simulink model "Longitudinal_Simulink_MaskedParameter_Stateflow_Virtual"  (Simulink 7.1)
settings: Solver=ode45  StartTime=0.0  StopTime=5.0  RelTol=1e-3
libraries: vrlib x2
settings Model: Creator=Meisel  LastModifiedBy=Meisel

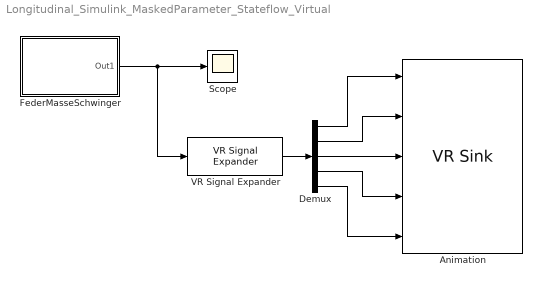
== system Longitudinal_Simulink_MaskedParameter_Stateflow_Virtual ==
  Animation : vrlib/VR Sink  SampleTime=0.01  ViewEnable=on  RemoteChange=off  RemoteView=on  FieldsWritten=m05.translation.3.1.double#m04.translation.3.1.double#m03.translation.3.1.double#m02.translation.3.1.double#m01.translation.3.1.double  WorldFileName=Massen_5.WRL  AutoView=off  VideoDimensions=[]  FigureProperties="{'Position', 'Name', 'Viewpoint', 'CameraBound', 'CameraDirection', 'CameraPosition', 'CameraUpVector', 'ZoomFactor', 'Antialiasing', 'Headlight', 'Lighting', 'NavPanel', 'StatusBar', 'ToolBar', 'Textures', 'Transparency', 'Wireframe', 'NavZones', 'NavMode', 'NavSpeed', 'Record2DCompressMethod', 'Record2DCompressQuality', 'Record2D', 'Record2DFileName', 'Record2DFPS'; [9.2000000000000000e+001  1.2400000000000000e+002  4.9100000000000000e+002  1.8200000000000000e+002], '', '_untitled_2', 'on', [5.2633573936155620e-001 -1.8738127758298598e-001 -8.2937262209581786e-001], [4.6106517249297135e-001  4.9665536299408264e-001 -9.6042888045995545e-001], [1.0040389152691827e-001  9.8228725778733783e-001 -1.5821125672619779e-001], [1.0000000000000000e+000], 'off', 'on', 'on', 'halfbar', 'off', 'on', 'on', 'on', 'off', 'off', 'examine', 'normal', 'auto', [7.5000000000000000e+001], 'off', '%f_anim_%n.avi', [1.5000000000000000e+001]}"
  Demux : Demux  Outputs=5
  FederMasseSchwinger : Subsystem  mask{k_init=1000, m=1, l0=1}
      mask prompts: k_init "Federkonstanten"; m "Massen"; l0 "Federlänge"
  Scope : Scope
      settings: TimeRange=5  YMin=1  YMax=5.5
  VR Signal Expander : vrlib/VR Signal Expander  SystemSampleTime=-1  outwidth=15  outidx=[13 10 7 4 1]
  wires:
  FederMasseSchwinger/1(Out1) -> Scope/1, VR Signal Expander/1
  VR Signal Expander/1 -> Demux/1
  Demux/1 -> Animation/1
  Demux/2 -> Animation/2
  Demux/3 -> Animation/3
  Demux/4 -> Animation/4
  Demux/5 -> Animation/5

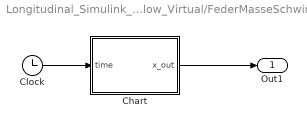
== system Longitudinal_Simulink_MaskedParameter_Stateflow_Virtual/FederMasseSchwinger ==
  Chart : Stateflow chart
  Clock : Clock
      settings: Decimation=10
  Out1 : Outport
  wires:
  Clock/1 -> Chart/1(time)
  Chart/1(x_out) -> Out1/1

== stateflow chart FederMasseSchwinger/Chart ==
  settings: updateMethod=CONTINUOUS
  state Schwinge
    during:
    // derivatives
    x_dot=v;
    v_dot=Acceleration();
    // output
    x_out=x;
    // Draw();
  (default) -> Schwinge : { InitCond(); }
  Schwinge -> Schwinge [order 1] : [ time >= 0.1 && x0==0 ]
      | { x0=0.25*l0; }
  Schwinge -> Schwinge [order 2] : [ time >= 2 && FederOK() ]
      | { FederReisst() }
  data: a function_output double size=n; f function_output boolean; n constant int32 =5; x local double size=n; v local double size=n; k local double size=n; m parameter double; l0 parameter double; time input double; x_out output double size=n; x0 local double; xend local double; k_init parameter double; k0 local double size=1
  data n settings: description=Anzahl der Massen
  data x settings: updateMethod=SF_CONTINUOUS_TIME_DATA  description=Position der Massen
  data v settings: updateMethod=SF_CONTINUOUS_TIME_DATA  description=Geschwindigkeit der Massen
  data k settings: description=Federkonstanten
  data m settings: description=Masse
  data l0 settings: description=Federlänge der entspannten Feder
  data time settings: description=Systemzeit
  data x_out settings: description=Positionen der Massen
  function InitCond:
    | function InitCond
    |     % Die k Massen auf die Startpositionen setzen.
    |     % Abstand zweier Massen: l0
    |     for i = 1:n
    |         x(i) = l0*i;  
    |         k(i) = k_init;
    |     end
    |    
    |     x0   = 0;        % Ort des Eingangspunktes
    |     xend = double(l0*(n+1));  % Ort des Endpunktes
    |     k0   = k_init;   % Federkonstante der ersten Feder
    | end
  function a  = Acceleration:
    | function a  = Acceleration
    |     
    |     % Achtung: Size des Rückgabeparameters a muss im 
    |     % ModelExplorer explizit auf n gesetzt werden !!!
    |     a=zeros(n,1);
    |     
    |     % Die erste und die letzte Masse müssen gesondert
    |     % behandelt werden
    |     a(1)=( -(x(1)-x0    -l0)*k0     + (x(2)-x(1)-l0)*k(1) ) / m;
    |     a(n)=( -(x(n)-x(n-1)-l0)*k(n-1) + (xend-x(n)-l0)*k(n) ) / m;    
    |     
    |     % Kraftwirikung zwischen den Massen 2 ... n-1
    |     for i=2:n-1
    |         a(i) = ( -(x(i)-x(i-1)-l0)*k(i-1) + (x(i+1)-x(i)-l0)*k(i) ) / m;
    |     end
  function f=FederOK:
    | function f=FederOK()
    |     f=true;      % Muss im ModelExplorer explizit
    |                  % auf Boolean gesetzt werden !
    |     if k(n)== 0  % Wenn k(n)==0, dann ist Feder defekt
    |         f=false;  
    |     end
    | end
  function FederReisst:
    | function FederReisst
    | % Feder defekt -> Federkonstante = 0
    |     k(n)=0; 
    | end
